simulink model "ExampleOrientation"  (Simulink 9.2)
settings: Solver=FixedStepDiscrete  StartTime=0.0  StopTime=inf  FixedStep=0.01  RelTol=1e-3  EnableMultiTasking=on
InitFcn:
  | % Set up script for the ExampleOrientation model.
  | 
  | % 3 Lines showing axes of model frame
  | % (ISO axis definitions since Matlab uses a right handed axis system by default)
  | localAxes_xpts = [1.5, 0, 0, 0, 0];
  | localAxes_ypts = [  0, 0, 1, 0, 0];
  | localAxes_zpts = [  0, 0, 0, 0, 1];
  | localAxes = [localAxes_xpts; localAxes_ypts; localAxes_zpts];
  | 
  | % Patch in the form of an arrow showing the world frame
  | % (ISO axis definition since Matlab uses a right handed axis system by default)
  | worldAxes_xpts = [-1  ,  0  ,  0, 1, 0, 0  , -1  ];
  | worldAxes_ypts = [-0.5, -0.5, -1, 0, 1, 0.5,  0.5];
  | worldAxes_zpts = [ 0  ,  0  ,  0, 0, 0, 0  ,  0  ];
  | worldAxes = [worldAxes_xpts; worldAxes_ypts; worldAxes_zpts];
  | 
  | % Prepare the Matlab figure showing the output
  | figure(1);
  | clf
  | 
  | subplot(2,1,1);
  | local_ax1 = plot3(localAxes_xpts, localAxes_ypts, localAxes_zpts, 'LineWidth', 2);
  | world_ax1 = patch(worldAxes_xpts, worldAxes_ypts, worldAxes_zpts, [1 0 0], 'FaceAlpha', 0.1);
  | axis([-2 2 -2 2 -2 2])
  | grid
  | 
  | subplot(2,1,2);
  | local_ax2 = plot3(localAxes_xpts, localAxes_ypts, localAxes_zpts, 'LineWidth', 2);
  | world_ax2 = patch(worldAxes_xpts, worldAxes_ypts, worldAxes_zpts, [1 0 0], 'FaceAlpha', 0.1);
  | axis([-2 2 -2 2 -2 2])
  | grid
  | text_h = text('Position',[0.5, 2, 3.5],'String','Roll: 0, Pitch: 0, Yaw: 0', 'FontSize', 18, 'FontWeight', 'bold');
libraries: simulink x7, rFproPhysicsLib x4
CloseFcn:
  | clear localAxes localAxes_xpts localAxes_ypts localAxes_zpts
  | clear worldAxes worldAxes_xpts worldAxes_ypts worldAxes_zpts
  | clear text_h local_ax1 world_ax1 local_ax2 world_ax2
  | close(figure(1))
settings Model: Creator=enewton  LastModifiedBy=SeanKavanagh
settings DataIOCC: SaveOutput=off  SaveTime=off
settings OptimizationCC: ExpressionDepthLimit=2147483647
settings DebuggingCC: SolverPrmCheckMsg=warning
settings RTWCC: TargetLang=C++

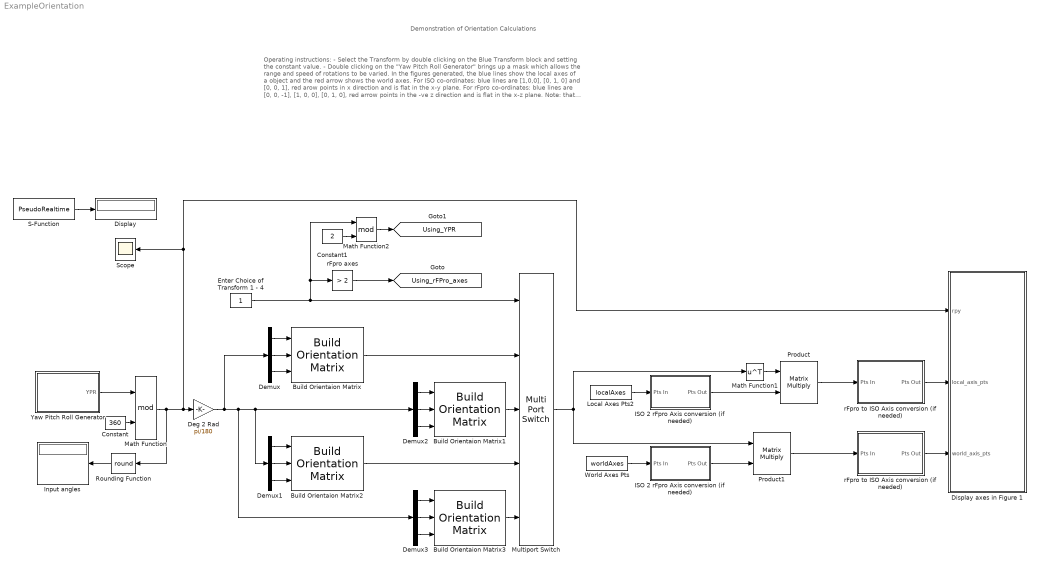
== system ExampleOrientation ==
  note: Demonstration of Orientation Calculations
  note: Operating instructions:
      |
      | - Select the Transform by double clicking on the Blue Transform block and setting the constant value.
      | - Double clicking on the "Yaw Pitch Roll Generator" brings up a mask which allows the range and speed of rotations to be varied.
      |
      | In the figures generated, the blue lines show the local axes of a object and the red arrow shows the world axes.
      |
      | For ISO co-ordinates: blue lines are [1,0,0], [0, 1, 0] and [0, 0, 1], red arow points in x direction and is flat in the x-y plane.
      | For rFpro co-ordinates: blue lines are [0, 0, -1], [1, 0, 0], [0, 1, 0], red arrow points in the -ve z direction and is flat in the x-z plane.
      |
      | Note: that since Matlab uses the ISO co-ordinate system, we convert to and from rFpro co-ordinates when working in the latter system,
      | so that the results can be displayed in the figure.
  Build Orientaion Matrix : rFproPhysicsLib/Build Orientation Matrix  ISOAxes=on  YPROrder=on
  Build Orientaion Matrix1 : rFproPhysicsLib/Build Orientation Matrix  ISOAxes=on  YPROrder=off
  Build Orientaion Matrix2 : rFproPhysicsLib/Build Orientation Matrix  ISOAxes=off  YPROrder=on
  Build Orientaion Matrix3 : rFproPhysicsLib/Build Orientation Matrix  ISOAxes=off  YPROrder=off
  Constant : Constant  Value=360
  Constant1 : Constant  Value=2
  Deg 2 Rad : Gain  Gain=pi/180
  Demux{,1..3} (4 alike) : Demux  Outputs=3
  Display : Display
  Display axes in Figure 1 : MATLAB Function  TreatAsAtomicUnit=on
  Enter Choice of Transform 1 - 4 : Constant
  ISO 2 rFpro Axis conversion (if needed) : Subsystem
  "ISO 2 rFpro Axis conversion (if needed) " : Subsystem
  Input angles : Display
  Local Axes Pts2 : Constant  Value=localAxes
  Math Function : Math  Operator=mod  SaturateOnIntegerOverflow=on
  Math Function1 : Math  Operator=transpose  SaturateOnIntegerOverflow=on
  Math Function2 : Math  Operator=mod  SaturateOnIntegerOverflow=on
  Multiport Switch : MultiPortSwitch  Inputs=4
  Product : Product  Multiplication=Matrix(*)  RndMeth=Zero
  Product1 : Product  Multiplication=Matrix(*)  RndMeth=Zero
  Rounding Function : Rounding  Operator=round
  S-Function : S-Function  FunctionName=PseudoRealtime  Parameters=0.01  SFunctionDeploymentMode=off  EnableBusSupport=off
  Scope : Scope
  World Axes Pts : Constant  Value=worldAxes
  Yaw Pitch Roll Generator : Subsystem  mask(Yaw, Pitch and Roll Generator){maxYaw=360 + 30, maxPitch=360 + 10, maxRoll=360 + 15, angleSpeed=1}
      mask prompts: maxYaw "Max Yaw (degrees)"; maxPitch "Max Pitch (degrees)"; maxRoll "Max Roll (degrees)"; angleSpeed "Speed"
      mask help:
      | Enter the maximum values for the roll, pitch and yaw and the
      | output will run from zero to the maximum of each in turn,
      | holding the last value for the other angles.
      |
      | Speed scales how fast the angles change (default is 1).
      |
      | The order in which each is increased is found using the "Using_YPR" goto signal.
  rFpro axes : simulink/Logic and Bit Operations/Compare To Constant  relop=>  const=2  OutDataTypeStr=boolean
  rFpro to ISO Axis conversion (if needed) : Subsystem
  "rFpro to ISO Axis conversion (if needed) " : Subsystem
  tag scope: Using_YPR=global, Using_rFPro_axes=global
  wires:
  Deg 2 Rad/1 -> Demux/1, Demux3/1, Demux1/1, Demux2/1
  Constant/1 -> Math Function/2
  Yaw Pitch Roll Generator/1(YPR) -> Math Function/1
  Math Function/1 -> Rounding Function/1, Deg 2 Rad/1, Scope/1, Display axes in Figure 1/1(rpy)
  S-Function/1 -> Display/1
  Math Function1/1 -> Product/1
  Enter Choice of Transform 1 - 4/1 -> Math Function2/1, rFpro axes/1, Multiport Switch/1
  Build Orientaion Matrix1/1 -> Multiport Switch/3
  Multiport Switch/1 -> Math Function1/1, Product1/1
  rFpro axes/1 -> [Using_rFPro_axes]
  ISO 2 rFpro Axis conversion (if needed)/1(Pts Out) -> Product/2
  rFpro to ISO Axis conversion (if needed)/1(Pts Out) -> Display axes in Figure 1/2(local_axis_pts)
  Build Orientaion Matrix3/1 -> Multiport Switch/5
  World Axes Pts/1 -> "ISO 2 rFpro Axis conversion (if needed) "/1(Pts In)
  "ISO 2 rFpro Axis conversion (if needed) "/1(Pts Out) -> Product1/2
  Local Axes Pts2/1 -> ISO 2 rFpro Axis conversion (if needed)/1(Pts In)
  Product1/1 -> "rFpro to ISO Axis conversion (if needed) "/1(Pts In)
  "rFpro to ISO Axis conversion (if needed) "/1(Pts Out) -> Display axes in Figure 1/3(world_axis_pts)
  Product/1 -> rFpro to ISO Axis conversion (if needed)/1(Pts In)
  Constant1/1 -> Math Function2/2
  Math Function2/1 -> [Using_YPR]
  Rounding Function/1 -> Input angles/1
  Build Orientaion Matrix/1 -> Multiport Switch/2
  Build Orientaion Matrix2/1 -> Multiport Switch/4
  Demux/2 -> Build Orientaion Matrix/2
  Demux/1 -> Build Orientaion Matrix/1
  Demux/3 -> Build Orientaion Matrix/3
  Demux1/1 -> Build Orientaion Matrix2/1
  Demux1/2 -> Build Orientaion Matrix2/2
  Demux1/3 -> Build Orientaion Matrix2/3
  Demux2/3 -> Build Orientaion Matrix1/3
  Demux2/2 -> Build Orientaion Matrix1/2
  Demux2/1 -> Build Orientaion Matrix1/1
  Demux3/1 -> Build Orientaion Matrix3/1
  Demux3/2 -> Build Orientaion Matrix3/2
  Demux3/3 -> Build Orientaion Matrix3/3

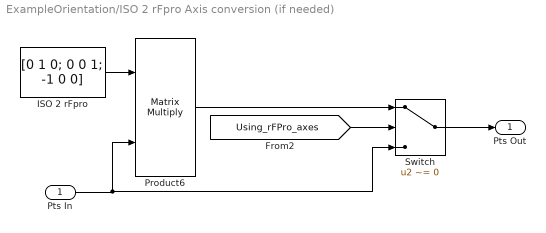
== system ExampleOrientation/ISO 2 rFpro Axis conversion (if needed) ==
  Pts In : Inport
  ISO 2 rFpro : Constant  Value=[0 1 0; 0 0 1; -1 0 0]
  Product6 : Product  Multiplication=Matrix(*)  RndMeth=Zero
  Switch : Switch  Criteria=u2 ~= 0  Threshold=2
  Pts Out : Outport
  wires:
  [Using_rFPro_axes] -> Switch/2
  Pts In/1 -> Switch/3, Product6/2
  ISO 2 rFpro/1 -> Product6/1
  Product6/1 -> Switch/1
  Switch/1 -> Pts Out/1

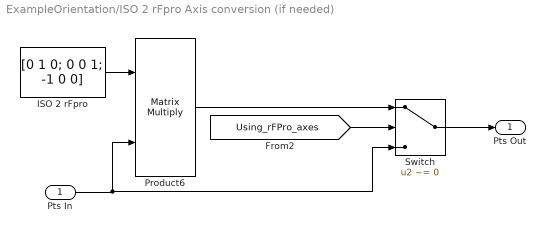
== system ExampleOrientation/ISO 2 rFpro Axis conversion (if needed)  ==
  Pts In : Inport
  ISO 2 rFpro : Constant  Value=[0 1 0; 0 0 1; -1 0 0]
  Product6 : Product  Multiplication=Matrix(*)  RndMeth=Zero
  Switch : Switch  Criteria=u2 ~= 0  Threshold=2
  Pts Out : Outport
  wires:
  Switch/1 -> Pts Out/1
  Product6/1 -> Switch/1
  ISO 2 rFpro/1 -> Product6/1
  Pts In/1 -> Product6/2, Switch/3
  [Using_rFPro_axes] -> Switch/2

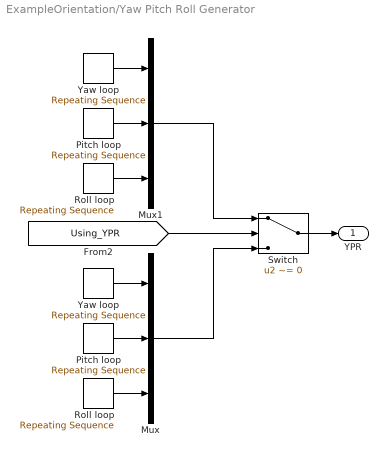
== system ExampleOrientation/Yaw Pitch Roll Generator ==
  Mux : Mux  Inputs=3
  Mux1 : Mux  Inputs=3
  Pitch loop : simulink/Sources/Repeating Sequence  rep_seq_t=angleSpeed * 0:8  rep_seq_y=maxPitch * [0 0 1 1 1 1 0 0 0]
  "Pitch loop " : simulink/Sources/Repeating Sequence  rep_seq_t=angleSpeed * 0:8  rep_seq_y=maxPitch * [0 0 0 1 1 0 0 0 0]
  Roll loop : simulink/Sources/Repeating Sequence  rep_seq_t=angleSpeed * 0:8  rep_seq_y=maxRoll * [0 0 0 1 1 0 0 0 0]
  "Roll loop " : simulink/Sources/Repeating Sequence  rep_seq_t=angleSpeed * 0:8  rep_seq_y=maxRoll * [0 0 1 1 1 1 0 0 0]
  Switch : Switch  Criteria=u2 ~= 0
  Yaw loop : simulink/Sources/Repeating Sequence  rep_seq_t=angleSpeed * 0:8  rep_seq_y=maxYaw * [0 1 1 1 1 1 1 0 0]
  "Yaw loop " : simulink/Sources/Repeating Sequence  rep_seq_t=angleSpeed * 0:8  rep_seq_y=maxYaw * [0 1 1 1 1 1 1 0 0]
  YPR : Outport
  wires:
  "Roll loop "/1 -> Mux/3
  "Yaw loop "/1 -> Mux/1
  "Pitch loop "/1 -> Mux/2
  [Using_YPR] -> Switch/2
  Roll loop/1 -> Mux1/3
  Yaw loop/1 -> Mux1/1
  Pitch loop/1 -> Mux1/2
  Mux1/1 -> Switch/1
  Mux/1 -> Switch/3
  Switch/1 -> YPR/1

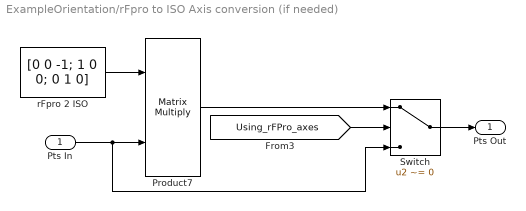
== system ExampleOrientation/rFpro to ISO Axis conversion (if needed) ==
  Pts In : Inport
  Product7 : Product  Multiplication=Matrix(*)  RndMeth=Zero
  Switch : Switch  Criteria=u2 ~= 0  Threshold=2
  rFpro 2 ISO : Constant  Value=[0 0 -1; 1 0 0; 0 1 0]
  Pts Out : Outport
  wires:
  rFpro 2 ISO/1 -> Product7/1
  Pts In/1 -> Switch/3, Product7/2
  Product7/1 -> Switch/1
  [Using_rFPro_axes] -> Switch/2
  Switch/1 -> Pts Out/1

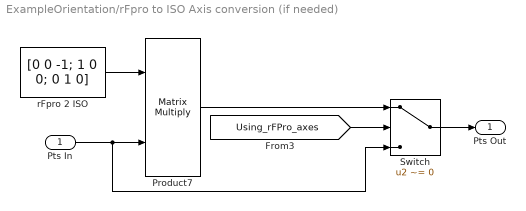
== system ExampleOrientation/rFpro to ISO Axis conversion (if needed)  ==
  Pts In : Inport
  Product7 : Product  Multiplication=Matrix(*)  RndMeth=Zero
  Switch : Switch  Criteria=u2 ~= 0  Threshold=2
  rFpro 2 ISO : Constant  Value=[0 0 -1; 1 0 0; 0 1 0]
  Pts Out : Outport
  wires:
  Switch/1 -> Pts Out/1
  [Using_rFPro_axes] -> Switch/2
  Product7/1 -> Switch/1
  Pts In/1 -> Product7/2, Switch/3
  rFpro 2 ISO/1 -> Product7/1

== matlab function Display axes in Figure 1 ==
  data: rpy input double; local_axis_pts input double; world_axis_pts input double
function fcn(rpy, local_axis_pts, world_axis_pts)
coder.extrinsic('evalin');
coder.extrinsic('sprintf');

subplot(2,1,2);
titleStr = sprintf('Yaw: %d, Pitch: %d, Roll: %d', round(rpy(1)), round(rpy(2)), round(rpy(3)));
set(evalin('base', 'text_h'), 'String', titleStr);

local_ax1_h = evalin('base', 'local_ax1');
world_ax2_h = evalin('base', 'world_ax2');
set(local_ax1_h, 'XData', local_axis_pts(1,:), 'YData', local_axis_pts(2,:), 'ZData', local_axis_pts(3,:));
set(world_ax2_h, 'XData', world_axis_pts(1,:), 'YData', world_axis_pts(2,:), 'ZData', world_axis_pts(3,:));
